simulink model "Pendulum_sim"  (R2015a)
settings: Solver=ode45  StartTime=0.0  StopTime=10.0  RelTol=1e-3
InitFcn:
  | m = 15;
  | g = 9.81;
  | L = 1.7;
  | b = 2.0;
  | Ts = 0.02;
libraries: simulink x1
settings Model: Creator=Logan  LastModifiedBy=Logan

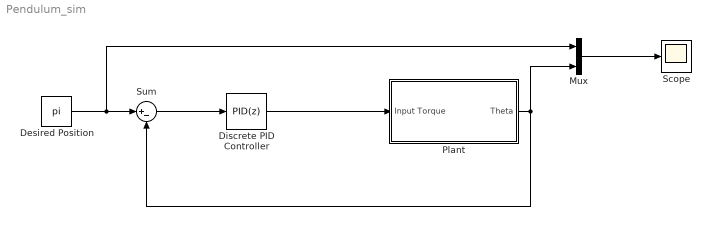
== system Pendulum_sim ==
  Desired Position : Constant  Value=pi  SampleTime=Ts
  Discrete PID Controller : simulink/Continuous/PID Controller  Controller=PID  TimeDomain=Discrete-time  SampleTime=0.01  IntegratorMethod=Forward Euler  FilterMethod=Forward Euler  Form=Parallel  UseFilter=off  ControllerParametersSource=internal  P=800  I=50  D=300  N=250  InitialConditionSource=internal  InitialConditionForIntegrator=0  InitialConditionForFilter=0  ExternalReset=none  LimitOutput=off  UpperSaturationLimit=inf  LowerSaturationLimit=-inf  LinearizeAsGain=off  AntiWindupMode=none  Kb=1  TrackingMode=off  Kt=1  PParamMin=[]  PParamMax=[]  IParamMin=[]  IParamMax=[]  DParamMin=[]  DParamMax=[]  NParamMin=[]  NParamMax=[]  KbParamMin=[]  KbParamMax=[]  KtParamMin=[]  KtParamMax=[]  POutMin=[]  POutMax=[]  IOutMin=[]  IOutMax=[]  DOutMin=[]  DOutMax=[]  NOutMin=[]  NOutMax=[]  KbOutMin=[]  KbOutMax=[]  KtOutMin=[]  KtOutMax=[]  IntegratorOutMin=[]  IntegratorOutMax=[]  FilterOutMin=[]  FilterOutMax=[]  SumOutMin=[]  SumOutMax=[]  SumI1OutMin=[]  SumI1OutMax=[]  SumI2OutMin=[]  SumI2OutMax=[]  SumI3OutMin=[]  SumI3OutMax=[]  SumDOutMin=[]  SumDOutMax=[]  SaturationOutMin=[]  SaturationOutMax=[]  IntegratorContinuousStateAttributes=''  IntegratorStateMustResolveToSignalObject=off  IntegratorRTWStateStorageClass=Auto  FilterContinuousStateAttributes=''  FilterStateMustResolveToSignalObject=off  FilterRTWStateStorageClass=Auto  DifferentiatorICPrevScaledInput=0  DifferentiatorOutMin=[]  DifferentiatorOutMax=[]
  Mux : Mux  Inputs=2
  Plant : Subsystem
  Scope : Scope
      settings: TimeRange=10  YMin=0  YMax=3
  Sum : Sum  Inputs=|+-
  wires:
  Discrete PID Controller/1 -> Plant/1(Input Torque)
  Plant/1(Theta) -> Sum/2, Mux/2
  Sum/1 -> Discrete PID Controller/1
  Desired Position/1 -> Mux/1, Sum/1
  Mux/1 -> Scope/1

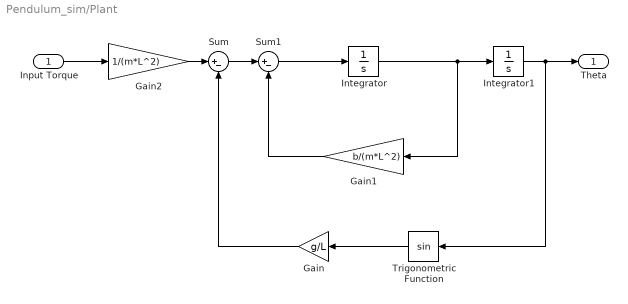
== system Pendulum_sim/Plant ==
  Input Torque : Inport
  Gain : Gain  Gain=g/L
  Gain1 : Gain  Gain=b/(m*L^2)
  Gain2 : Gain  Gain=1/(m*L^2)
  Integrator : Integrator
  Integrator1 : Integrator
  Sum : Sum  Inputs=|+-
  Sum1 : Sum  Inputs=|+-
  Trigonometric Function : Trigonometry
  Theta : Outport
  wires:
  Gain/1 -> Sum/2
  Gain1/1 -> Sum1/2
  Sum/1 -> Sum1/1
  Sum1/1 -> Integrator/1
  Input Torque/1 -> Gain2/1
  Gain2/1 -> Sum/1
  Integrator/1 -> Integrator1/1, Gain1/1
  Integrator1/1 -> Theta/1, Trigonometric Function/1
  Trigonometric Function/1 -> Gain/1
